simulink model "model_biquad_wfa"  (R2020b)
settings: Solver=VariableStepAuto  StartTime=0.0  StopTime=1  RelTol=1e-3
values from neighbouring files (symbols this model uses):
  in_cos = 2*cos(2*pi*k/N)    [compute_constants.m]    (also in signat_to_test_generate.m = -2*cos(2*pi*k/N))
  Ts = 1e-3    (= 0.001)    [compute_constants.m]    (also in signat_to_test_generate.m)
  Wkn = -exp(-j*2*pi*k/N)    [compute_constants.m]    (also in signat_to_test_generate.m)
undefined symbols (not defined in the file or in its folder): dfilt
libraries: simulink x2, dsparch4 x1
settings Model: Creator=pablo  LastModifiedBy=pablo

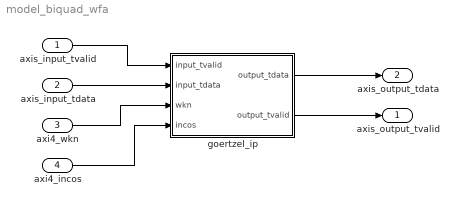
== system model_biquad_wfa ==
  axis_input_tvalid : Inport
  axis_input_tdata : Inport  Port=2
  axi4_wkn : Inport  Port=3
  axi4_incos : Inport  Port=4
  goertzel_ip : Subsystem
  axis_output_tvalid : Outport
  axis_output_tdata : Outport  Port=2
  wires:
  goertzel_ip/1(output_tdata) -> axis_output_tdata/1
  axis_input_tvalid/1 -> goertzel_ip/1(input_tvalid)
  axis_input_tdata/1 -> goertzel_ip/2(input_tdata)
  goertzel_ip/2(output_tvalid) -> axis_output_tvalid/1
  axi4_wkn/1 -> goertzel_ip/3(wkn)
  axi4_incos/1 -> goertzel_ip/4(incos)

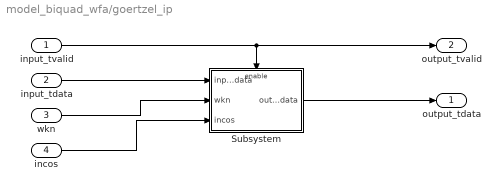
== system model_biquad_wfa/goertzel_ip ==
  input_tvalid : Inport  OutDataTypeStr=boolean
  input_tdata : Inport  Port=2  OutDataTypeStr=fixdt(1,32,16)
  wkn : Inport  Port=3  OutDataTypeStr=fixdt(1,32,16)
  incos : Inport  Port=4  OutDataTypeStr=fixdt(1,32,16)
  Subsystem : Subsystem
  output_tdata : Outport
  output_tvalid : Outport  Port=2  InitialOutput=0
  wires:
  input_tvalid/1 -> output_tvalid/1, Subsystem/Enable
  input_tdata/1 -> Subsystem/1(input_data)
  wkn/1 -> Subsystem/2(wkn)
  incos/1 -> Subsystem/3(incos)
  Subsystem/1(output_data) -> output_tdata/1

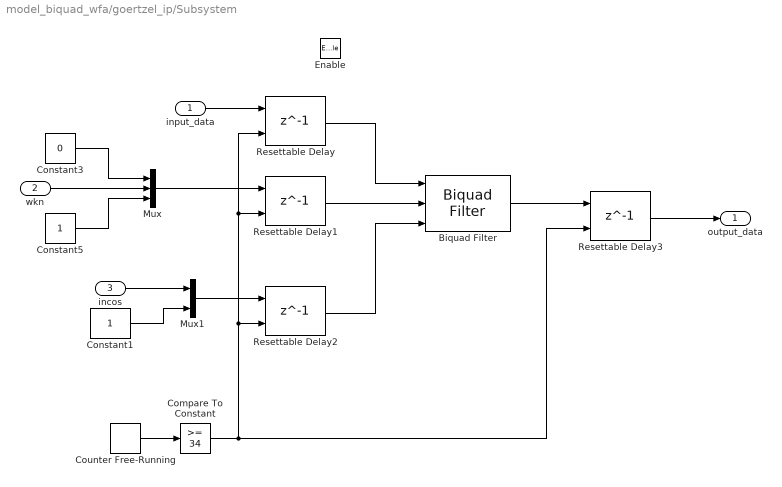
== system model_biquad_wfa/goertzel_ip/Subsystem ==
  input_data : Inport  OutDataTypeStr=fixdt(1,32,16)  SampleTime=Ts
  wkn : Inport  Port=2  OutDataTypeStr=fixdt(1,32,16)  SampleTime=Ts
  incos : Inport  Port=3  OutDataTypeStr=fixdt(1,32,16)  SampleTime=Ts
  Enable : EnablePort
  Biquad Filter : dsparch4/Biquad Filter  FilterSource=Input port(s)  CoeffSource=Specify via dialog  FilterObject=dfilt.df2tsos([1 0.3 0.4],[1 0.1 0.2])  IIRFiltStruct=Direct form II transposed  BiQuadCoeffs=[0 1 real(Wkn) 1 -in_cos 1]  ScaleValues=1  IC=0  ICnum=0  ICden=0  a0Flag=Warning  optimizeScaleValues=on  ScaleValueMode=Assume all are unity and optimize  roundingMode=Floor  overflowMode=off  scaleValueFracLength=14  denProdOutputFracLength=30  denAccumFracLength=30  secondMemoryFracLength=15
      settings: SourceProductName=DSP System Toolbox
  Compare To Constant : simulink/Logic and Bit Operations/Compare To Constant  relop=>=  const=34  OutDataTypeStr=boolean
  Constant1 : Constant  OutDataTypeStr=fixdt(1,32,16)
  Constant3 : Constant  Value=0  OutDataTypeStr=fixdt(1,32,16)
  Constant5 : Constant  OutDataTypeStr=fixdt(1,32,16)
  Counter Free-Running : simulink/Sources/Counter Free-Running  NumBits=6  tsamp=-1
  Mux : Mux  Inputs=3
  Mux1 : Mux  Inputs=2
  Resettable Delay{,1..3} (4 alike) : Delay  DelayLength=1  ExternalReset=Level
      settings: InputPortMap=u0,r5
  output_data : Outport  InitialOutput=0
  wires:
  Constant3/1 -> Mux/1
  Constant5/1 -> Mux/3
  Constant1/1 -> Mux1/2
  wkn/1 -> Mux/2
  incos/1 -> Mux1/1
  input_data/1 -> Resettable Delay/1
  Resettable Delay/1 -> Biquad Filter/1
  Mux/1 -> Resettable Delay1/1
  Resettable Delay1/1 -> Biquad Filter/2
  Mux1/1 -> Resettable Delay2/1
  Resettable Delay2/1 -> Biquad Filter/3
  Counter Free-Running/1 -> Compare To Constant/1
  Compare To Constant/1 -> Resettable Delay3/2, Resettable Delay/2, Resettable Delay1/2, Resettable Delay2/2
  Biquad Filter/1 -> Resettable Delay3/1
  Resettable Delay3/1 -> output_data/1
